simulink model "squareroot_funcblock"  (R2019b)
settings: Solver=VariableStepAuto  StartTime=0.0  StopTime=1  RelTol=1e-3
settings Model: Creator=kanth  LastModifiedBy=kanth

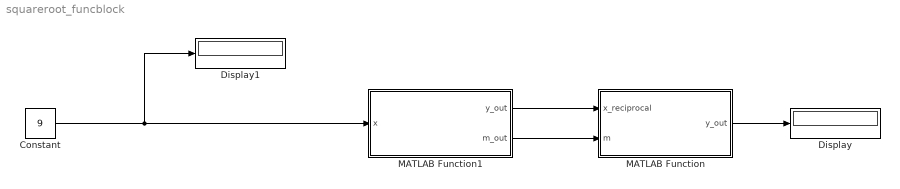
== system squareroot_funcblock ==
  Constant : Constant  Value=9  OutDataTypeStr=fixdt(1,16,8)  SampleTime=-1
  Display : Display
      settings: Decimation=1000
  Display1 : Display
      settings: Format=binary (Stored Integer)  Decimation=1000
  MATLAB Function : MATLAB Function  TreatAsAtomicUnit=on
  MATLAB Function1 : MATLAB Function  TreatAsAtomicUnit=on
  wires:
  MATLAB Function/1(y_out) -> Display/1
  MATLAB Function1/1(y_out) -> MATLAB Function/1(x_reciprocal)
  MATLAB Function1/2(m_out) -> MATLAB Function/2(m)
  Constant/1 -> Display1/1, MATLAB Function1/1(x)

== matlab function squareroot_funcblock/MATLAB Function1 ==
  data: x input; y_out output; m_out output
function [y_out,m_out] = reciprocal(x)
%x=3;
    x_comp = x*(2^8);
    x_bin = dec2bin(x_comp);
    b = fi(0,true,16,8,'bin','0100000000000000');
    a = fi(x,true,16,8);
    count = 0;
    c = 0;
    while(c==0)
        count = count+1;
        bit = bitand(a,b);
        if (bit == 0)
            b = bitsrl(b,1);
        else
            c = 1;
        end
    end

    m = 8-count;
    if (m < 0)
        m = 0;
    end

    y = 2^(-m);

    err = 1;
    while(err>0.001)
    %Iterative eq
        %disp(y)
        y_k = y*(2-x*y);
        err = abs(y_k - y);
        y = y_k;
    end
    y_out = y;
    m_out = m;
end

== matlab function squareroot_funcblock/MATLAB Function ==
  data: x_reciprocal input; y_out output; m input
function y_out  = squareroot(x_reciprocal,m)
    
    y = 2^(floor(m/2));
    err = 1;
    while(err>0.01)
        %Iterative eq
         %disp(y)
        y_k = (y*0.5)*(3-((y^2)*x_reciprocal));
        err = abs(y_k - y);
        y = y_k;
    end
    y_out = y;
end
